simulink model "myModel2"  (Simulink 6.6)
settings: Solver=ode45  StartTime=0.0  StopTime=8  RelTol=1e-3
libraries: simulink x1
settings Model: Creator=Controls  LastModifiedBy=Controls
settings RTWCC: IncludeERTFirstTime=on

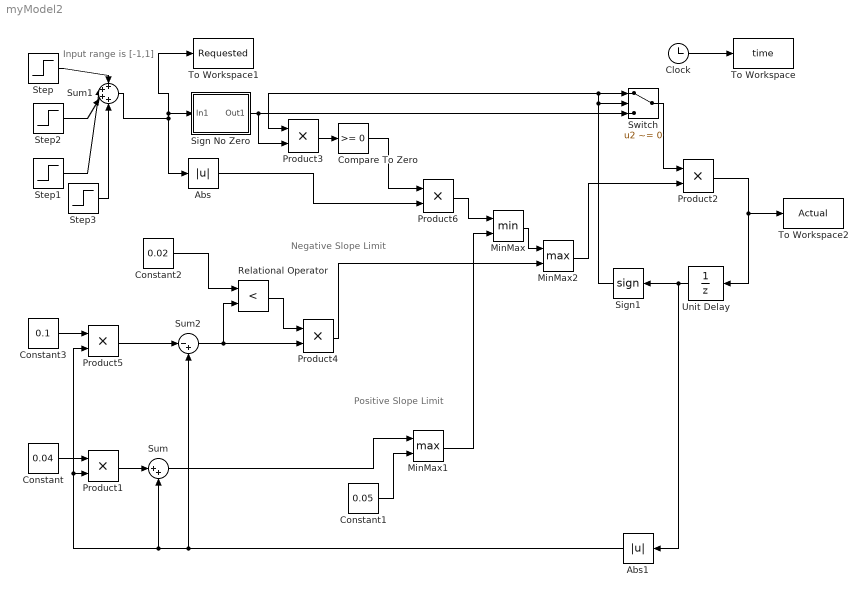
== system myModel2 ==
  note: Input range is [-1,1]
  note: Negative Slope Limit
  note: Positive Slope Limit
  Abs : Abs
  Abs1 : Abs  Orientation=left
  Clock : Clock
      settings: Decimation=10
  Compare To Zero : simulink/Logic and Bit Operations/Compare To Zero  SystemSampleTime=-1  relop=>=  LogicOutDataTypeMode=uint8  ZeroCross=off
  Constant : Constant  Value=0.04
  Constant1 : Constant  Value=0.05
  Constant2 : Constant  Value=0.02
  Constant3 : Constant  Value=0.1
  MinMax : MinMax  Inputs=2
  MinMax1 : MinMax  Function=max  Inputs=2
  MinMax2 : MinMax  Function=max  Inputs=2
  Product{1..6} (6 alike) : Product  RndMeth=Zero
  Relational Operator : RelationalOperator  Operator=<  LogicOutDataTypeMode=Boolean
  Sign No Zero : Subsystem
  Sign1 : Signum  Orientation=left
  Step : Step  SampleTime=0
  Step1 : Step  Time=3.2  SampleTime=0
  Step2 : Step  Time=3  After=-2  SampleTime=0
  Step3 : Step  Time=5  After=-0.2  SampleTime=0
  Sum : Sum  Inputs=|++
  Sum1 : Sum  Inputs=4
  Sum2 : Sum  Inputs=|-+
  Switch : Switch  Criteria=u2 ~= 0
  To Workspace : ToWorkspace  VariableName=time  SampleTime=-1  SaveFormat=Array
  To Workspace1 : ToWorkspace  VariableName=Requested  SampleTime=-1  SaveFormat=Array
  To Workspace2 : ToWorkspace  VariableName=Actual  SampleTime=-1  SaveFormat=Array
  Unit Delay : UnitDelay  Orientation=left  SampleTime=1/200
  wires:
  Constant/1 -> Product1/1
  Product1/1 -> Sum/1
  Unit Delay/1 -> Sign1/1, Abs1/1
  Abs1/1 -> Sum/2, Product1/2, Product5/2, Sum2/2
  MinMax1/1 -> MinMax/2
  Sum1/1 -> Sign No Zero/1(In1), To Workspace1/1, Abs/1
  MinMax2/1 -> Product2/2
  MinMax/1 -> MinMax2/1
  Sum/1 -> MinMax1/1
  Sum2/1 -> Relational Operator/2, Product4/2
  Product4/1 -> MinMax2/2
  Clock/1 -> To Workspace/1
  Constant1/1 -> MinMax1/2
  Relational Operator/1 -> Product4/1
  Constant2/1 -> Relational Operator/1
  Constant3/1 -> Product5/1
  Product5/1 -> Sum2/1
  Sign1/1 -> Switch/2, Switch/1, Product3/1
  Sign No Zero/1(Out1) -> Switch/3, Product3/2
  Switch/1 -> Product2/1
  Product2/1 -> Unit Delay/1, To Workspace2/1
  Product3/1 -> Compare To Zero/1
  Product6/1 -> MinMax/1
  Abs/1 -> Product6/2
  Compare To Zero/1 -> Product6/1
  Step/1 -> Sum1/1
  Step1/1 -> Sum1/2
  Step2/1 -> Sum1/3
  Step3/1 -> Sum1/4

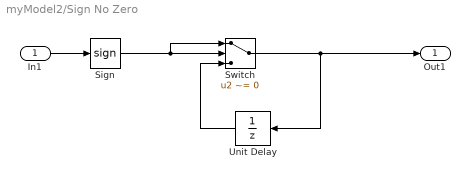
== system myModel2/Sign No Zero ==
  In1 : Inport
  Sign : Signum
  Switch : Switch  Criteria=u2 ~= 0
  Unit Delay : UnitDelay  Orientation=left  X0=1  SampleTime=1/200
  Out1 : Outport
  wires:
  In1/1 -> Sign/1
  Sign/1 -> Switch/2, Switch/1
  Unit Delay/1 -> Switch/3
  Switch/1 -> Out1/1, Unit Delay/1
